simulink model "Delta1"  (R2020b)
settings: Solver=VariableStepAuto  StartTime=0.0  StopTime=10.0  RelTol=1e-3
undefined symbols (not defined in the file): Matlab_version, Output_File, Output_file_n, Plant_inputs_num, Plant_outputs_num, RecurDyn, RecurDyn_controltimestep, RecurDyn_model, RecurDyn_model_n, X, Y, Z
libraries: sm_lib x7, nesl_utility x4
settings Model: Creator=23801  LastModifiedBy=23801

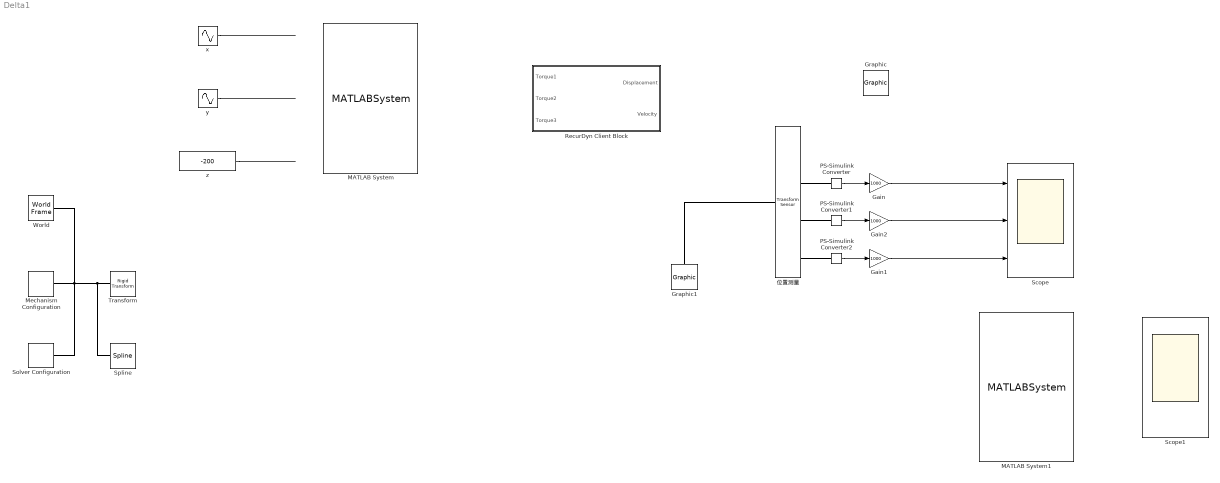
== system Delta1 ==
  Gain : Gain  Gain=1000
  Gain1 : Gain  Gain=1000
  Gain2 : Gain  Gain=1000
  Graphic : sm_lib/Body Elements/Graphic  GraphicType=Marker  MarkerShape=Sphere  MarkerSize=10  GraphicVisPropType=SimpleVisualProperties  GraphicDiffuseColor=[0.5 0.5 0.5]  GraphicSpecularColor=[0.5 0.5 0.5 1.0]  GraphicAmbientColor=[0.15 0.15 0.15 1.0]  GraphicEmissiveColor=[0.0 0.0 0.0 1.0]  GraphicShininess=75  GraphicOpacity=1.0
  Graphic1 : sm_lib/Body Elements/Graphic  GraphicType=Marker  MarkerShape=Sphere  MarkerSize=10  GraphicVisPropType=SimpleVisualProperties  GraphicDiffuseColor=[0.5 0.5 0.5]  GraphicSpecularColor=[0.5 0.5 0.5 1.0]  GraphicAmbientColor=[0.15 0.15 0.15 1.0]  GraphicEmissiveColor=[0.0 0.0 0.0 1.0]  GraphicShininess=75  GraphicOpacity=1.0
  MATLAB System : MATLABSystem
  MATLAB System1 : MATLABSystem
  Mechanism Configuration : sm_lib/Utilities/Mechanism Configuration  UniformGravity=Constant  GravityVector=[0 0 -9.80665]  GravityVectorUnits=m/s^2  GravityUnits=m/s^2  LinearizationDelta=0.001  JointModeTransitionNonlinearIterations=2
  PS-Simulink Converter : nesl_utility/PS-Simulink Converter  PhysicalDomain=network_engine_domain  SubClassName=ps_output  LeftPortType=input  RightPortType=output  PseudoPeriodic=off  Frequencies=[]  Unit=inherit  AffineConversion=off
  PS-Simulink Converter1 : nesl_utility/PS-Simulink Converter  PhysicalDomain=network_engine_domain  SubClassName=ps_output  LeftPortType=input  RightPortType=output  PseudoPeriodic=off  Frequencies=[]  Unit=inherit  AffineConversion=off
  PS-Simulink Converter2 : nesl_utility/PS-Simulink Converter  PhysicalDomain=network_engine_domain  SubClassName=ps_output  LeftPortType=input  RightPortType=output  PseudoPeriodic=off  Frequencies=[]  Unit=inherit  AffineConversion=off
  RecurDyn Client Block : Subsystem
      mask Display: image(imread('RecurDyn_IF3x_Client.jpg'))
  Scope : Scope  NumInputPorts=3
  Scope1 : Scope  NumInputPorts=3
  Solver Configuration : nesl_utility/Solver Configuration  PhysicalDomain=network_engine_domain  SubClassName=solver  LeftPortType=input  RightPortType=generic  Tones=[]  Harmonics=[]  SimulateNoise=off  Profile=off  UseLocalSampling=off  EnableSwitchedLinearOptims=on  FrequencyDomain=off  UseCCode=off  RelTol=0.001  AbsTol=1e-06  MinStep=1e-09  ToWorkspace=off  RevertToSquareIcSolve=off  NumHomotopyIterations=100  PhasorMode=off  PhasorModeNumHarmonics=1  DoDC=off  ResidualTolerance=1e-09  UseLocalSolver=off  LocalSolverChoice=NE_BACKWARD_EULER_ADVANCER  LocalSolverSampleTime=0.001  DoFixedCost=off  MaxNonlinIter=3  MaxModeIter=2  ComputeImpulses=off  ImpulseIterations=2  LinearAlgebra=auto  EquationFormulation=NE_TIME_EF  DelaysMemoryBudget=1024  AutomaticFiltering=on  FilteringTimeConstant=0.001  PartitionStorageMethod=AS_NEEDED  PartitionMemoryBudget=1024  PartitionMethod=ROBUST
  Spline : sm_lib/Curves and Surfaces/Spline  GraphicAmbientColor=[0.15 0.15 0.15 1.0]  GraphicDiffuseColor=[0.0 0.0 0.0]  DataPoints=[6 -2 9;-6 5 -4;-6 -7 9;6 0 -4;-3 6 9;-3 -8 -4]  DataPointsUnits=m  GraphicEmissiveColor=[0.0 0.0 0.0 1.0]  EndConditionType=Closed  MarkerShape=Sphere  MarkerSize=10  GraphicType=FromGeometry  GraphicOpacity=1.0  GraphicShininess=75  GraphicSpecularColor=[0.5 0.5 0.5 1.0]  GraphicVisPropType=SimpleVisualProperties
  Transform : sm_lib/Frames and Transforms/Rigid Transform  TranslationMethod=None  TranslationStandardOffset=0  TranslationLengthUnit=m  TranslationStandardAxis=+Z  TranslationCartesianOffset=[0 0 0]  TranslationROffset=0  TranslationROffsetUnits=m  TranslationZOffset=0  TranslationZOffsetUnits=m  TranslationThetaOffset=0  TranslationThetaOffsetUnits=deg  RotationMethod=None  RotationAngleUnits=deg  RotationStandardAxis=+Z  RotationAngle=0.0  RotationArbitraryAxis=[0 0 1]  FollAlignAxisA=+X  BaseAlignAxisA=+Y  FollAlignAxisB=+Y  BaseAlignAxisB=+Z  RotationSequenceAxes=FollowerAxes  RotationSequence=XYX  RotationSequenceAngles=[0 0 0]  RotationSequenceAnglesUnits=deg  RotationMatrix=[1 0 0; 0 1 0; 0 0 1]
  World : sm_lib/Frames and Transforms/World Frame
  x : Sin  SampleTime=0
  y : Sin  SampleTime=0
  z : Constant  Value=-200
  位置测量 : sm_lib/Frames and Transforms/Transform Sensor  Description=3  MeasurementFrame=World  SenseAngle=off  SenseAxis=off  SenseAngle1=off  SenseAngle2=off  SenseAngle3=off  SenseQ=off  SenseR=off  SenseOmegaX=off  SenseOmegaY=off  SenseOmegaZ=off  SenseOmega1=off  SenseOmega2=off  SenseOmega3=off  SenseQDot=off  SenseRDot=off  SenseAlphaX=off  SenseAlphaY=off  SenseAlphaZ=off  SenseAlpha1=off  SenseAlpha2=off  SenseAlpha3=off  SenseQDDot=off  SenseRDDot=off  SenseX=on  SenseY=on  SenseZ=on  SenseRad=off  SenseAzim=off  SenseDist=off  SenseInc=off  SenseXDot=off  SenseYDot=off  SenseZDot=off  SenseRadDot=off  SenseAzimDot=off  SenseDistDot=off  SenseIncDot=off  SenseXDDot=off  SenseYDDot=off  SenseZDDot=off  SenseRadDDot=off  SenseAzimDDot=off  SenseDistDDot=off  SenseIncDDot=off
  wires:
  x/1 -> ?
  y/1 -> ?
  z/1 -> ?
  Gain/1 -> Scope/1
  Gain2/1 -> Scope/2
  Gain1/1 -> Scope/3
  PS-Simulink Converter/1 -> Gain/1
  PS-Simulink Converter1/1 -> Gain2/1
  PS-Simulink Converter2/1 -> Gain1/1
  connections:
  Transform/LConn1 -- Solver Configuration/RConn1 -- World/RConn1 -- Mechanism Configuration/RConn1 -- Spline/LConn1
  Graphic1/RConn1 -- 位置测量/LConn1
  位置测量/RConn2 -- PS-Simulink Converter/LConn1
  位置测量/RConn3 -- PS-Simulink Converter1/LConn1
  位置测量/RConn4 -- PS-Simulink Converter2/LConn1

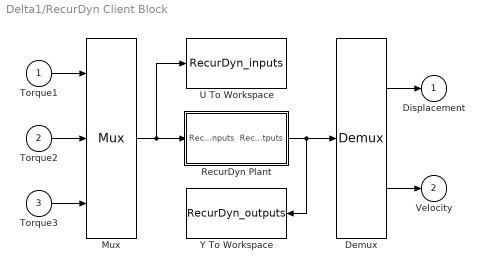
== system Delta1/RecurDyn Client Block ==
  Torque1 : Inport
  Torque2 : Inport  Port=2
  Torque3 : Inport  Port=3
  Demux : Demux  Outputs=2
      settings: DisplayOption=none
  Mux : Mux  Inputs=3
  RecurDyn Plant : Subsystem  mask(Recurdyn/Plant){RecurDyn_model_name=RecurDyn_model, Output_File_Name_=Output_File, RecurDyn_=RecurDyn, Matlab_version_=Matlab_version, RecurDyn_controltimestep_=RecurDyn_controltimestep, RecurDyn_step_=100, Waitingtime=1000, RecurDyn_static_=off, RecurDyn_show_=on, RecurDyn_ani_=on, Create_Output_Folder_=off}
      mask prompts: Output_File_Name_ "Output File Name"; RecurDyn_ "RecurDyn_install_directory"; Matlab_version_ "Matlab version"; RecurDyn_controltimestep_ "Sampling period"; RecurDyn_step_ "RecurDyn_step"; Waitingtime "Waiting time"; RecurDyn_static_ "Static analysis"; RecurDyn_show_ "RecurDyn_show"; RecurDyn_ani_ "RecurDyn_animation"; Create_Output_Folder_ "Create Output Folder"
      mask help:
      | Simulate any Recurdyn Dynamics Model in Recurdyn/Solver
      | Plant inputs and Plant outputs are transfered every sampling time
      | Here, sampling time is determined by sampling period (Control time step)
      mask Display: disp( 'Dynamic Model' )
  U To Workspace : ToWorkspace  VariableName=RecurDyn_inputs
  Y To Workspace : ToWorkspace  VariableName=RecurDyn_outputs
  Displacement : Outport
  "Velocity    " : Outport  Port=2
  wires:
  RecurDyn Plant/1(RecurDyn_outputs) -> Demux/1, Y To Workspace/1
  Mux/1 -> RecurDyn Plant/1(" RecurDyn_inputs"), U To Workspace/1
  Demux/1 -> Displacement/1
  Demux/2 -> "Velocity    "/1
  Torque1/1 -> Mux/1
  Torque2/1 -> Mux/2
  Torque3/1 -> Mux/3

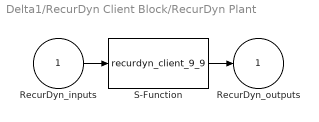
== system Delta1/RecurDyn Client Block/RecurDyn Plant ==
  " RecurDyn_inputs" : Inport
  S-Function : S-Function  FunctionName=recurdyn_client_9_9  Parameters=RecurDyn_controltimestep_,RecurDyn_model_name,RecurDyn_,RecurDyn_static_,RecurDyn_step_,RecurDyn_show_,RecurDyn_ani_,Matlab_version_,RecurDyn_model_n,Plant_inputs_num,Plant_outputs_num,Waitingtime,Create_Output_Folder_,Output_File_Name_,Output_file_n  SFunctionDeploymentMode=off  EnableBusSupport=off
  RecurDyn_outputs : Outport  InitialOutput=0
  wires:
  S-Function/1 -> RecurDyn_outputs/1
  " RecurDyn_inputs"/1 -> S-Function/1
